simulink model "ALKEC_smlk"  (R2015b)
settings: Solver=VariableStepAuto  SolverMode=SingleTasking  StartTime=0.0  StopTime=1000  MaxStep=1  MinStep=0.0001  RelTol=1e-3
values from neighbouring files (symbols this model uses):
  A_cell = 0.25    [ALKEC_begin.m]
  c_cw = 4.18e03    (= 4180)    [ALKEC_cellstack.m]    (also in ALKEC_data.m)
  C_th = 625e03    (= 625000)    [ALKEC_data.m]
  DeltaP = (p_an - p_atm) / eta_p    [ALKEC_data.m]
  eta_ACDC = 0.95    [ALKEC_data.m]
  F = 96485    [ALKEC_begin.m]
  f1 = 2.50    (= 2.5)    [ALKEC_data.m]
  f2 = 0.97    [ALKEC_data.m]
  h_cond = 250    [ALKEC_data.m]
  h_conv = 0.97    [ALKEC_data.m]
  m_cw = 0.0850    (= 0.085)    [ALKEC_cellstack.m]    (also in ALKEC_data.m = 0.25)
  M_H2 = 2.01588    [ALKEC_cellstack.m]    (also in ALKEC_data.m)
  M_H2O = 18.01528    [ALKEC_cellstack.m]    (also in ALKEC_data.m)
  M_O2 = 31.9988    [ALKEC_cellstack.m]    (also in ALKEC_data.m)
  N_cell = 90    [ALKEC_begin.m]
  P_gamma = 2.5e03    (= 2500)    [ALKEC_data.m]
  p_H2avg = (p_H2in + p_H2out) / 2    [ALKEC_data.m]
  p_H2Oavg = (p_H2Oin + p_H2Oout) / 2    [ALKEC_data.m]
  p_O2avg = (p_O2in + p_O2out) / 2    [ALKEC_data.m]
  R = 8.314    [ALKEC_begin.m]
  r1 = 3.53855e-04    (= 0.000353855)    [ALKEC_data.m]
  r2 = -3.02150e-06    (= -3.0215e-06)    [ALKEC_data.m]
  R_th = 0.167    [ALKEC_data.m]
  s = 0.22396    [ALKEC_data.m]
  T = 80 + 273.15    (= 353.15)    [ALKEC_begin.m]
  T0 = T_a    [ALKEC_data.m]
  t1 = 2.73093    [ALKEC_data.m]
  t2 = -2.40447e02    (= -240.447)    [ALKEC_data.m]
  t3 = 5.99576e03    (= 5995.76)    [ALKEC_data.m]
  T_a = 25    [ALKEC_begin.m]
  T_amb = 25    [ALKEC_begin.m]    (also in ALKEC_data.m = T_a + 273.15)
  T_cwin = 20 + 0    (= 20)    [ALKEC_cellstack.m]    (also in ALKEC_data.m)
  T_des = T - 273.15    [ALKEC_data.m]
  tau_E = 2.00    (= 2)    [ALKEC_data.m]
  tau_p = 0.5    [ALKEC_data.m]
  tau_th = C_th * R_th    [ALKEC_cellstack.m]    (also in ALKEC_data.m = 104375)
  U = polyval(polU, I(1))    [ALKEC_data.m]
  v_H2 = 0.08988e03    (= 89.88)    [ALKEC_cellstack.m]    (also in ALKEC_data.m)
  v_H240 = 3.1777e03    (= 3177.7)    [ALKEC_data.m]
  v_H2O = 999.97e03    (= 999970)    [ALKEC_cellstack.m]    (also in ALKEC_data.m = 999700)
  v_O2 = 1.308e03    (= 1308)    [ALKEC_cellstack.m]    (also in ALKEC_data.m)
  v_O240 = 52.876e03    (= 52876)    [ALKEC_data.m]
  V_tn = 1.48    [ALKEC_cellstack.m]    (also in ALKEC_data.m)
  VS_H2 = 40    [ALKEC_data.m]
  VS_O2 = 20    [ALKEC_data.m]
  zeta = 1    [ALKEC_data.m]
undefined symbols (not defined in the file or in its folder): magnitude
settings Model: Creator=gapaolo  LastModifiedBy=gapaolo
settings DataIOCC: SaveFormat=Array
settings OptimizationCC: BlockReduction=off  BooleanDataType=off
settings DebuggingCC: AlgebraicLoopMsg=none  SaveWithParameterizedLinksMsg=none  UnderspecifiedInitializationDetection=Classic  MergeDetectMultiDrivingBlocksExec=none  SignalResolutionControl=TryResolveAllWithWarning
settings HardwareCC: ProdBitPerPointer=32  ProdLargestAtomicFloat=None  ProdIntDivRoundTo=Undefined  ProdEndianess=Unspecified  ProdWordSize=32  ProdHWDeviceType=32-bit Generic  TargetUnknown=on
settings GRTTargetCC: GeneratePreprocessorConditionals=Disable all
settings ConfigComp: CovModelRefEnable=Off  CovSFcnEnable=off

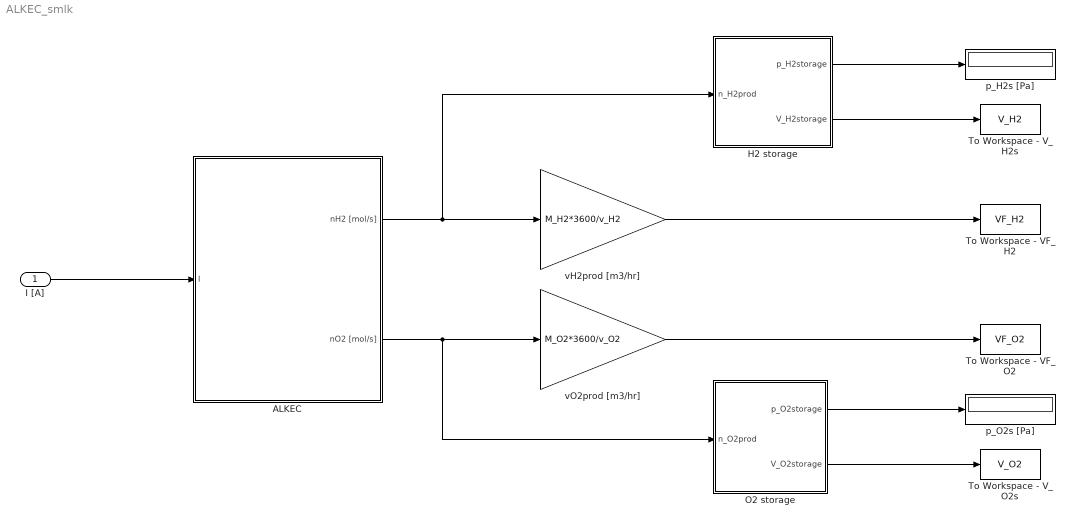
== system ALKEC_smlk ==
  I [A] : Inport
  ALKEC : Subsystem
  H2 storage : Subsystem
  O2 storage : Subsystem
  To Workspace - VF_H2 : ToWorkspace  VariableName=VF_H2  SaveFormat=Timeseries  SampleTime=-1
  To Workspace - VF_O2 : ToWorkspace  VariableName=VF_O2  SaveFormat=Timeseries  SampleTime=-1
  To Workspace - V_H2s : ToWorkspace  VariableName=V_H2  SaveFormat=Timeseries  SampleTime=-1
  To Workspace - V_O2s : ToWorkspace  VariableName=V_O2  SaveFormat=Timeseries  SampleTime=-1
  p_H2s [Pa] : Display
  p_O2s [Pa] : Display
  vH2prod [m3/hr] : Gain  Gain=M_H2*3600/v_H2
  vO2prod [m3/hr] : Gain  Gain=M_O2*3600/v_O2
  wires:
  I [A]/1 -> ALKEC/1(I)
  H2 storage/1(p_H2storage) -> p_H2s [Pa]/1
  ALKEC/2(nO2 [mol/s]) -> O2 storage/1(n_O2prod), vO2prod [m3/hr]/1
  O2 storage/1(p_O2storage) -> p_O2s [Pa]/1
  H2 storage/2(V_H2storage) -> To Workspace - V_H2s/1
  O2 storage/2(V_O2storage) -> To Workspace - V_O2s/1
  vH2prod [m3/hr]/1 -> To Workspace - VF_H2/1
  vO2prod [m3/hr]/1 -> To Workspace - VF_O2/1
  ALKEC/1(nH2 [mol/s]) -> H2 storage/1(n_H2prod), vH2prod [m3/hr]/1

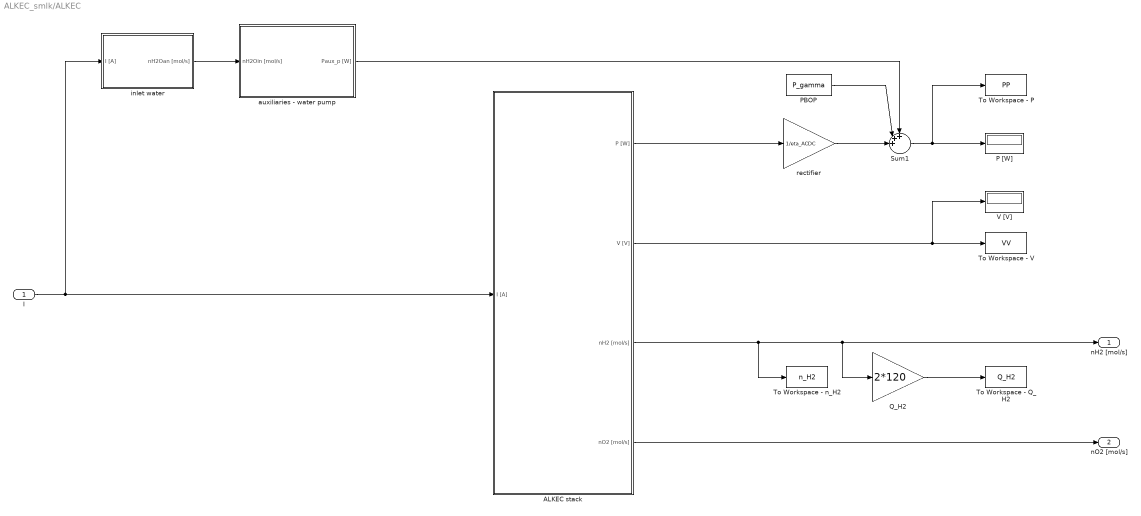
== system ALKEC_smlk/ALKEC ==
  I : Inport
  ALKEC stack : Subsystem
  P [W] : Display
  PBOP : Constant  Value=P_gamma
  Q_H2 : Gain  Gain=2*120
  Sum1 : Sum  Inputs=+++||
  To Workspace - P : ToWorkspace  VariableName=PP  SaveFormat=Timeseries  SampleTime=-1
  To Workspace - Q_H2 : ToWorkspace  VariableName=Q_H2  SaveFormat=Timeseries  SampleTime=-1
  To Workspace - V : ToWorkspace  VariableName=VV  SaveFormat=Timeseries  SampleTime=-1
  To Workspace - n_H2 : ToWorkspace  VariableName=n_H2  SaveFormat=Timeseries  SampleTime=-1
  V [V] : Display
  auxiliaries - water pump : Subsystem
  inlet water : Subsystem
  rectifier : Gain  Gain=1/eta_ACDC
  nH2 [mol/s] : Outport
  nO2 [mol/s] : Outport  Port=2
  wires:
  ALKEC stack/2(V [V]) -> To Workspace - V/1, V [V]/1
  I/1 -> inlet water/1(I [A]), ALKEC stack/1(I [A])
  ALKEC stack/1(P [W]) -> rectifier/1
  inlet water/1("nH2Oan [mol/s] ") -> auxiliaries - water pump/1(nH2Oin [mol/s])
  rectifier/1 -> Sum1/3
  Sum1/1 -> To Workspace - P/1, P [W]/1
  PBOP/1 -> Sum1/2
  auxiliaries - water pump/1(Paux_p [W]) -> Sum1/1
  ALKEC stack/4(nO2 [mol/s]) -> nO2 [mol/s]/1
  ALKEC stack/3(nH2 [mol/s]) -> To Workspace - n_H2/1, Q_H2/1, nH2 [mol/s]/1
  Q_H2/1 -> To Workspace - Q_H2/1

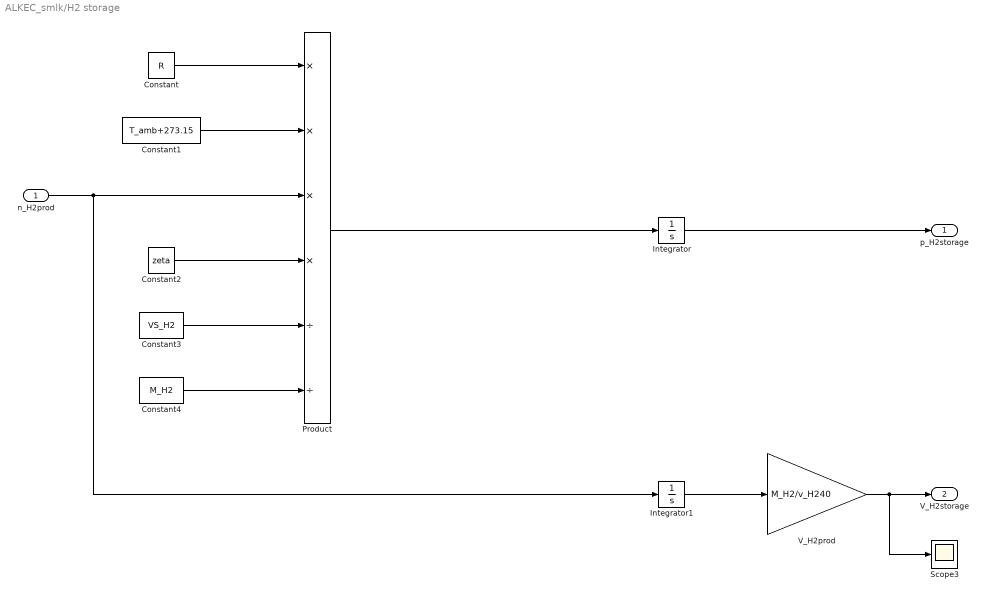
== system ALKEC_smlk/H2 storage ==
  n_H2prod : Inport
  Constant : Constant  Value=R
  Constant1 : Constant  Value=T_amb+273.15
  Constant2 : Constant  Value=zeta
  Constant3 : Constant  Value=VS_H2
  Constant4 : Constant  Value=M_H2
  Integrator : Integrator  InitialCondition=101325
  Integrator1 : Integrator
  Product : Product  Inputs=****//
  Scope3 : Scope
  V_H2prod : Gain  Gain=M_H2/v_H240
  p_H2storage : Outport
  V_H2storage : Outport  Port=2
  wires:
  n_H2prod/1 -> Integrator1/1, Product/3
  Constant/1 -> Product/1
  Constant1/1 -> Product/2
  Constant2/1 -> Product/4
  Constant3/1 -> Product/5
  Constant4/1 -> Product/6
  Product/1 -> Integrator/1
  Integrator/1 -> p_H2storage/1
  Integrator1/1 -> V_H2prod/1
  V_H2prod/1 -> Scope3/1, V_H2storage/1

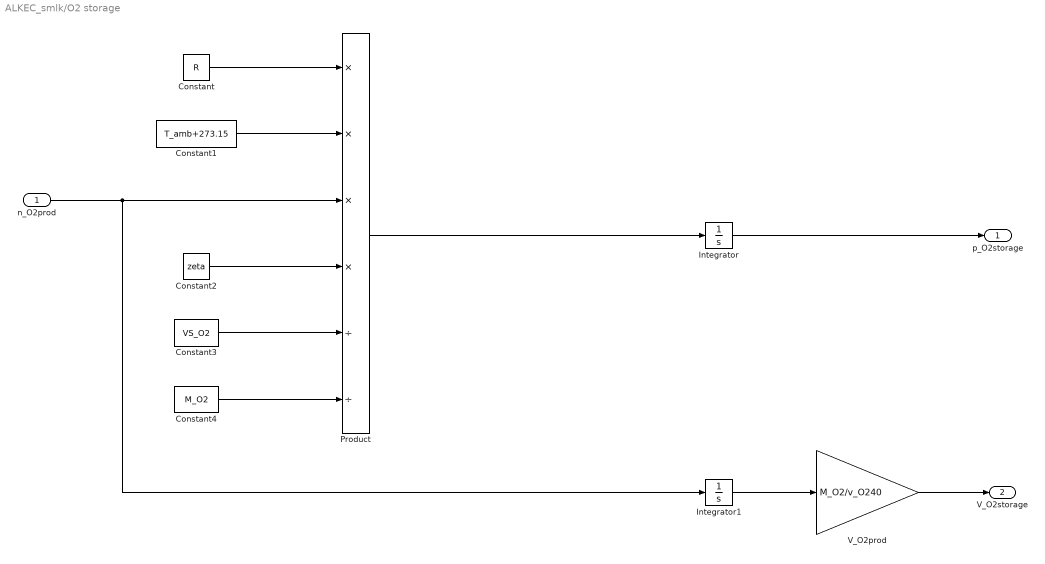
== system ALKEC_smlk/O2 storage ==
  n_O2prod : Inport
  Constant : Constant  Value=R
  Constant1 : Constant  Value=T_amb+273.15
  Constant2 : Constant  Value=zeta
  Constant3 : Constant  Value=VS_O2
  Constant4 : Constant  Value=M_O2
  Integrator : Integrator  InitialCondition=101325
  Integrator1 : Integrator
  Product : Product  Inputs=****//
  V_O2prod : Gain  Gain=M_O2/v_O240
  p_O2storage : Outport
  V_O2storage : Outport  Port=2
  wires:
  n_O2prod/1 -> Integrator1/1, Product/3
  Constant/1 -> Product/1
  Constant1/1 -> Product/2
  Constant2/1 -> Product/4
  Constant3/1 -> Product/5
  Constant4/1 -> Product/6
  Product/1 -> Integrator/1
  Integrator/1 -> p_O2storage/1
  Integrator1/1 -> V_O2prod/1
  V_O2prod/1 -> V_O2storage/1

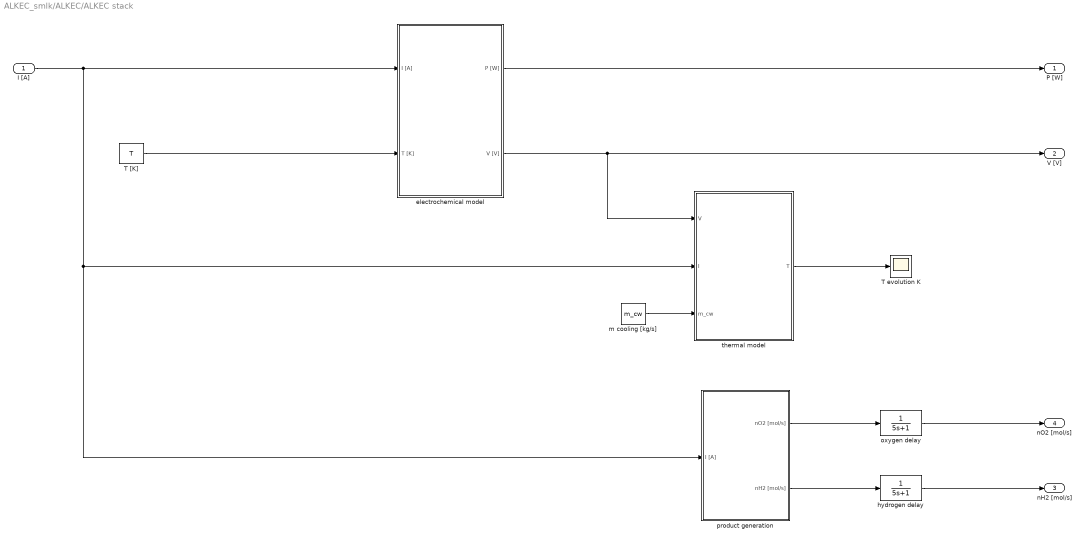
== system ALKEC_smlk/ALKEC/ALKEC stack ==
  I [A] : Inport
  T [K] : Constant  Value=T
  T evolution K : Scope
  electrochemical model : Subsystem
  hydrogen delay : TransferFcn  Denominator=[5 1]
  m cooling [kg/s] : Constant  Value=m_cw
  oxygen delay : TransferFcn  Denominator=[5 1]
  product generation : Subsystem
  thermal model : Subsystem
  P [W] : Outport
  V [V] : Outport  Port=2
  nH2 [mol/s] : Outport  Port=3
  nO2 [mol/s] : Outport  Port=4
  wires:
  m cooling [kg/s]/1 -> thermal model/3(m_cw)
  electrochemical model/2(V [V]) -> V [V]/1, thermal model/1(V)
  thermal model/1(T) -> T evolution K/1
  electrochemical model/1(P [W]) -> P [W]/1
  I [A]/1 -> product generation/1(I [A]), thermal model/2(I), electrochemical model/1(I [A])
  T [K]/1 -> electrochemical model/2(T [K])
  oxygen delay/1 -> nO2 [mol/s]/1
  hydrogen delay/1 -> nH2 [mol/s]/1
  product generation/1(nO2 [mol/s]) -> oxygen delay/1
  product generation/2(nH2 [mol/s]) -> hydrogen delay/1

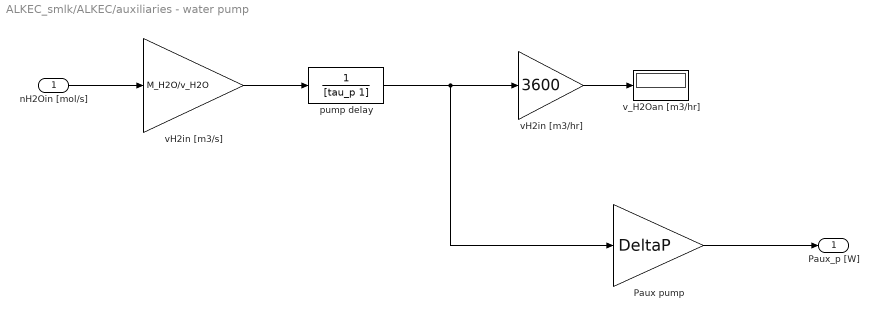
== system ALKEC_smlk/ALKEC/auxiliaries - water pump ==
  nH2Oin [mol/s] : Inport
  Paux pump : Gain  Gain=DeltaP
  pump delay : TransferFcn  Denominator=[tau_p 1]
  vH2in [m3/hr] : Gain  Gain=3600
  vH2in [m3/s] : Gain  Gain=M_H2O/v_H2O
  v_H2Oan [m3/hr] : Display
  Paux_p [W] : Outport
  wires:
  vH2in [m3/s]/1 -> pump delay/1
  vH2in [m3/hr]/1 -> v_H2Oan [m3/hr]/1
  Paux pump/1 -> Paux_p [W]/1
  nH2Oin [mol/s]/1 -> vH2in [m3/s]/1
  pump delay/1 -> vH2in [m3/hr]/1, Paux pump/1

== system ALKEC_smlk/ALKEC/inlet water ==
  I [A] : Inport
  Faraday efficiency : Subsystem
  I*eta_F : Product
  n_H2Ocons1 : Gain  Gain=N_cell/(2*F*U)
  "nH2Oan [mol/s] " : Outport
  wires:
  Faraday efficiency/2(I [A]) -> I*eta_F/2
  Faraday efficiency/1(eta_F) -> I*eta_F/1
  I*eta_F/1 -> n_H2Ocons1/1
  n_H2Ocons1/1 -> "nH2Oan [mol/s] "/1
  I [A]/1 -> Faraday efficiency/1(I)

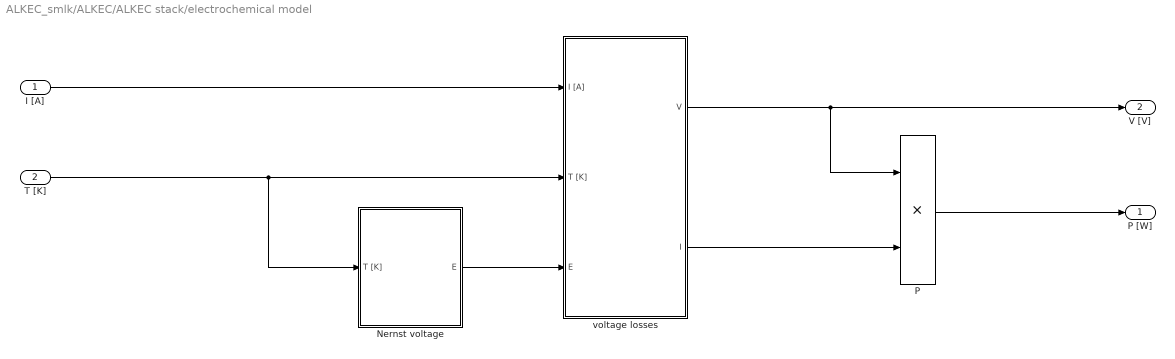
== system ALKEC_smlk/ALKEC/ALKEC stack/electrochemical model ==
  I [A] : Inport
  T [K] : Inport  Port=2
  Nernst voltage : Subsystem
  P : Product
  "voltage losses " : Subsystem
  P [W] : Outport
  V [V] : Outport  Port=2
  wires:
  I [A]/1 -> "voltage losses "/1("I [A] ")
  "voltage losses "/1(V) -> P/1, V [V]/1
  P/1 -> P [W]/1
  T [K]/1 -> "voltage losses "/2(T [K]), Nernst voltage/1(T [K])
  "voltage losses "/2(I) -> P/2
  Nernst voltage/1(E) -> "voltage losses "/3(E)

== system ALKEC_smlk/ALKEC/ALKEC stack/product generation ==
  I [A] : Inport
  Faraday efficiency : Subsystem
  I*eta_F : Product
  n_H2 : Gain  Gain=N_cell/(2*F)
  n_O2 : Gain  Gain=N_cell/(4*F)
  nO2 [mol/s] : Outport
  nH2 [mol/s] : Outport  Port=2
  wires:
  n_H2/1 -> nH2 [mol/s]/1
  n_O2/1 -> nO2 [mol/s]/1
  I [A]/1 -> Faraday efficiency/1(I)
  Faraday efficiency/2(I [A]) -> I*eta_F/2
  Faraday efficiency/1(eta_F) -> I*eta_F/1
  I*eta_F/1 -> n_O2/1, n_H2/1

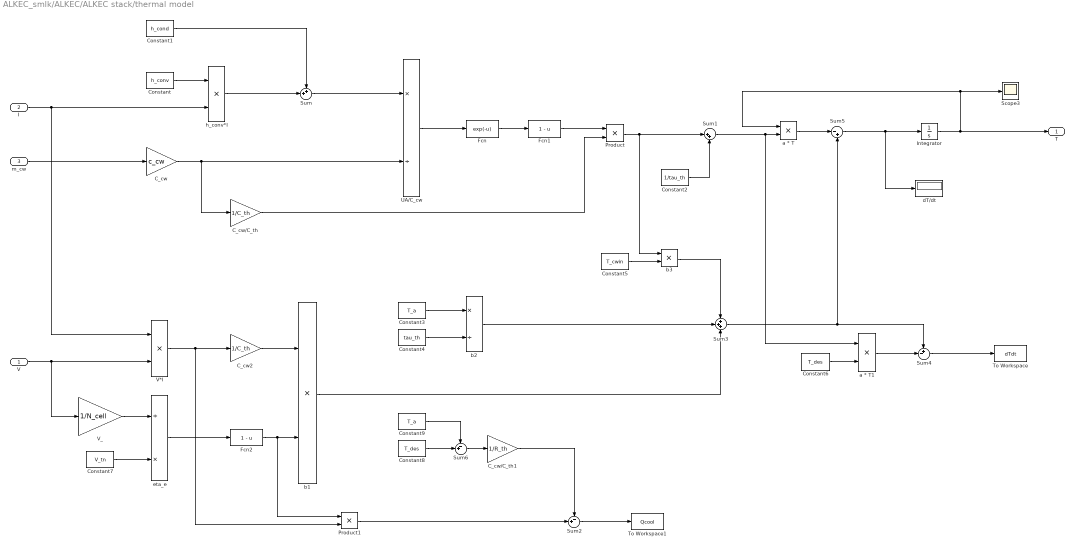
== system ALKEC_smlk/ALKEC/ALKEC stack/thermal model ==
  V : Inport
  I : Inport  Port=2
  m_cw : Inport  Port=3
  C_cw : Gain  Gain=c_cw
  C_cw/C_th : Gain  Gain=1/C_th
  C_cw/C_th1 : Gain  Gain=1/R_th
  C_cw2 : Gain  Gain=1/C_th
  Constant : Constant  Value=h_conv
  Constant1 : Constant  Value=h_cond
  Constant2 : Constant  Value=1/tau_th
  Constant3 : Constant  Value=T_a
  Constant4 : Constant  Value=tau_th
  Constant5 : Constant  Value=T_cwin
  Constant6 : Constant  Value=T_des
  Constant7 : Constant  Value=V_tn
  Constant8 : Constant  Value=T_des
  Constant9 : Constant  Value=T_a
  Fcn : Fcn  Expr=exp(-u)
  Fcn1 : Fcn  Expr=1 - u
  Fcn2 : Fcn  Expr=1 - u
  Integrator : Integrator  InitialCondition=T0
  Product : Product
  Product1 : Product
  Scope3 : Scope
  Sum : Sum  Inputs=++|
  Sum1 : Sum  Inputs=|++
  Sum2 : Sum  Inputs=-+|
  Sum3 : Sum  Inputs=+++
  Sum4 : Sum  Inputs=+-|
  Sum5 : Sum  Inputs=|-+
  Sum6 : Sum  Inputs=-+|
  To Workspace : ToWorkspace  VariableName=dTdt  SaveFormat=Timeseries  SampleTime=-1
  To Workspace1 : ToWorkspace  VariableName=Qcool  SaveFormat=Timeseries  SampleTime=-1
  UA/C_cw : Product  Inputs=*/
  V*I : Product
  V_ : Gain  Gain=1/N_cell
  a * T : Product
  a * T1 : Product
  b1 : Product
  b2 : Product  Inputs=*/
  b3 : Product
  dT/dt : Display
  eta_e : Product  Inputs=/*
  h_conv*I : Product
  T : Outport
  wires:
  I/1 -> V*I/1, h_conv*I/2
  Constant/1 -> h_conv*I/1
  h_conv*I/1 -> Sum/2
  Constant1/1 -> Sum/1
  Sum/1 -> UA/C_cw/1
  m_cw/1 -> C_cw/1
  UA/C_cw/1 -> Fcn/1
  Fcn/1 -> Fcn1/1
  C_cw/1 -> UA/C_cw/2, C_cw/C_th/1
  Fcn1/1 -> Product/1
  C_cw/C_th/1 -> Product/2
  Product/1 -> b3/1, Sum1/1
  Constant2/1 -> Sum1/2
  C_cw2/1 -> b1/1
  Constant3/1 -> b2/1
  Constant4/1 -> b2/2
  Constant5/1 -> b3/2
  b3/1 -> Sum3/1
  b2/1 -> Sum3/2
  V_/1 -> eta_e/1
  Constant7/1 -> eta_e/2
  eta_e/1 -> Fcn2/1
  Sum5/1 -> dT/dt/1, Integrator/1
  a * T/1 -> Sum5/1
  Sum1/1 -> a * T1/1, a * T/2
  Integrator/1 -> a * T/1, Scope3/1, T/1
  b1/1 -> Sum3/3
  Sum3/1 -> Sum4/1, Sum5/2
  Constant6/1 -> a * T1/2
  Sum4/1 -> To Workspace/1
  a * T1/1 -> Sum4/2
  Product1/1 -> Sum2/2
  Constant8/1 -> Sum6/2
  Constant9/1 -> Sum6/1
  Sum6/1 -> C_cw/C_th1/1
  C_cw/C_th1/1 -> Sum2/1
  Sum2/1 -> To Workspace1/1
  V*I/1 -> Product1/2, C_cw2/1
  Fcn2/1 -> Product1/1, b1/2
  V/1 -> V*I/2, V_/1

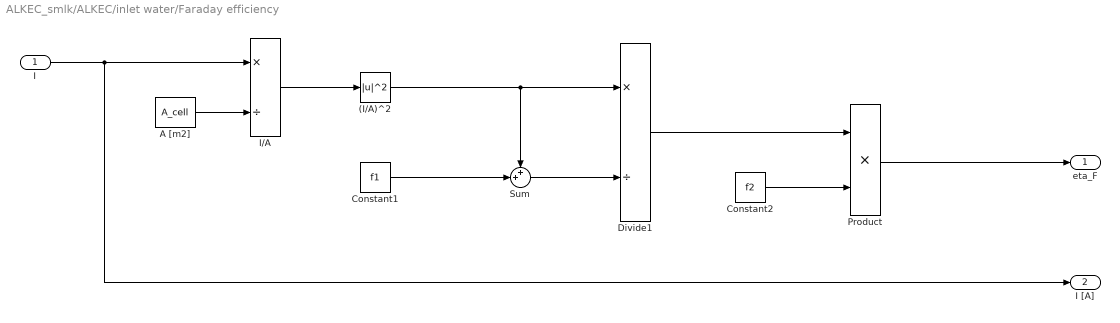
== system ALKEC_smlk/ALKEC/inlet water/Faraday efficiency ==
  I : Inport
  (I/A)^2 : Math  Operator=magnitude^2  SaturateOnIntegerOverflow=on
  A [m2] : Constant  Value=A_cell
  Constant1 : Constant  Value=f1
  Constant2 : Constant  Value=f2
  Divide1 : Product  Inputs=*/
  I/A : Product  Inputs=*/
  Product : Product
  Sum : Sum  Inputs=++|
  eta_F : Outport
  I [A] : Outport  Port=2
  wires:
  A [m2]/1 -> I/A/2
  I/1 -> I [A]/1, I/A/1
  I/A/1 -> (I/A)^2/1
  (I/A)^2/1 -> Sum/1, Divide1/1
  Constant1/1 -> Sum/2
  Sum/1 -> Divide1/2
  Divide1/1 -> Product/1
  Constant2/1 -> Product/2
  Product/1 -> eta_F/1

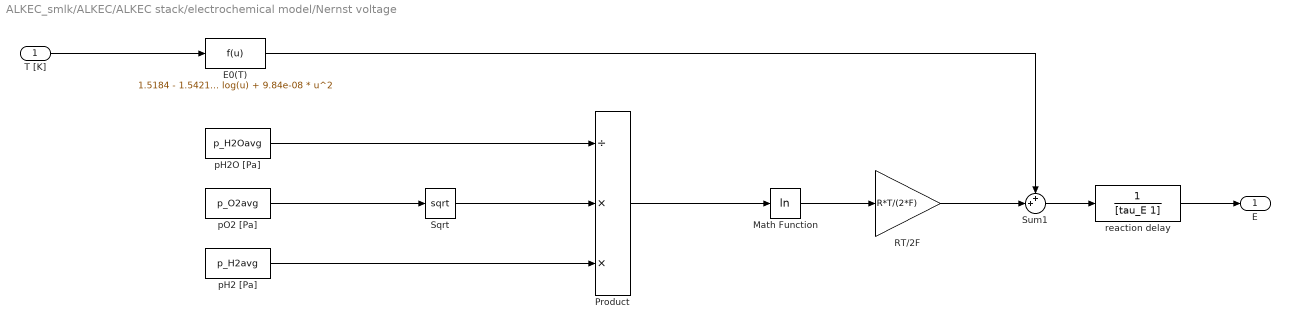
== system ALKEC_smlk/ALKEC/ALKEC stack/electrochemical model/Nernst voltage ==
  T [K] : Inport
  E0(T) : Fcn  Expr=1.5184 - 1.5421e-03 * u + 9.523e-05 * u * log(u) + 9.84e-08 * u^2
  Math Function : Math  Operator=log  SaturateOnIntegerOverflow=on
  Product : Product  Inputs=/**
  RT/2F : Gain  Gain=R*T/(2*F)
  Sqrt : Sqrt  SaturateOnIntegerOverflow=on
  Sum1 : Sum  Inputs=++|
  pH2 [Pa] : Constant  Value=p_H2avg
  pH2O [Pa] : Constant  Value=p_H2Oavg
  pO2 [Pa] : Constant  Value=p_O2avg
  reaction delay : TransferFcn  Denominator=[tau_E 1]
  E : Outport
  wires:
  RT/2F/1 -> Sum1/2
  E0(T)/1 -> Sum1/1
  Sum1/1 -> reaction delay/1
  Sqrt/1 -> Product/2
  Product/1 -> Math Function/1
  Math Function/1 -> RT/2F/1
  T [K]/1 -> E0(T)/1
  pH2O [Pa]/1 -> Product/1
  pH2 [Pa]/1 -> Product/3
  pO2 [Pa]/1 -> Sqrt/1
  reaction delay/1 -> E/1

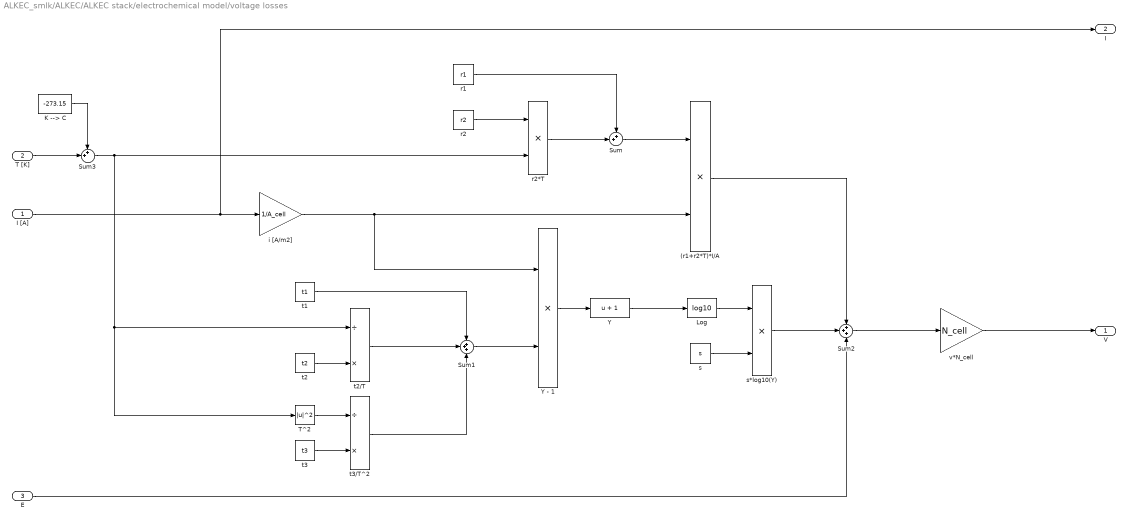
== system ALKEC_smlk/ALKEC/ALKEC stack/electrochemical model/voltage losses  ==
  "I [A] " : Inport
  T [K] : Inport  Port=2
  E : Inport  Port=3
  (r1+r2*T)*I/A : Product  Inputs=**
  K --> C : Constant  Value=-273.15
  Log : Math  Operator=log10  SaturateOnIntegerOverflow=on
  Sum : Sum  Inputs=++|
  Sum1 : Sum  Inputs=+++
  Sum2 : Sum  Inputs=+++
  Sum3 : Sum  Inputs=++|
  T^2 : Math  Operator=magnitude^2  SaturateOnIntegerOverflow=on
  Y : Fcn  Expr=u + 1
  Y - 1 : Product  Inputs=**
  i [A/m2] : Gain  Gain=1/A_cell
  r1 : Constant  Value=r1
  r2 : Constant  Value=r2
  r2*T : Product  Inputs=**
  s : Constant  Value=s
  s*log10(Y) : Product  Inputs=**
  t1 : Constant  Value=t1
  t2 : Constant  Value=t2
  t2/T : Product  Inputs=/*
  t3 : Constant  Value=t3
  t3/T^2 : Product  Inputs=/*
  v*N_cell : Gain  Gain=N_cell
  V : Outport
  I : Outport  Port=2
  wires:
  E/1 -> Sum2/3
  "I [A] "/1 -> I/1, i [A/m2]/1
  v*N_cell/1 -> V/1
  r2/1 -> r2*T/1
  r2*T/1 -> Sum/2
  r1/1 -> Sum/1
  Sum/1 -> (r1+r2*T)*I/A/1
  i [A/m2]/1 -> Y - 1/1, (r1+r2*T)*I/A/2
  t2/1 -> t2/T/2
  t3/1 -> t3/T^2/2
  t2/T/1 -> Sum1/2
  t1/1 -> Sum1/1
  t3/T^2/1 -> Sum1/3
  Y - 1/1 -> Y/1
  Y/1 -> Log/1
  s/1 -> s*log10(Y)/2
  Log/1 -> s*log10(Y)/1
  s*log10(Y)/1 -> Sum2/2
  (r1+r2*T)*I/A/1 -> Sum2/1
  Sum2/1 -> v*N_cell/1
  T^2/1 -> t3/T^2/1
  Sum1/1 -> Y - 1/2
  Sum3/1 -> T^2/1, t2/T/1, r2*T/2
  T [K]/1 -> Sum3/2
  K --> C/1 -> Sum3/1

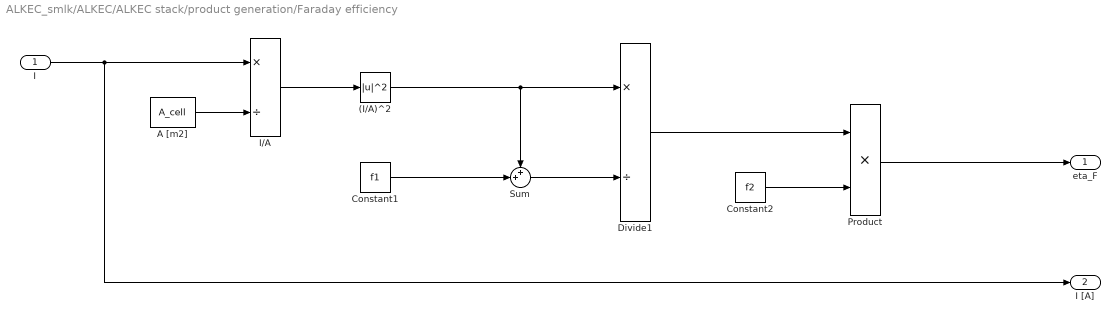
== system ALKEC_smlk/ALKEC/ALKEC stack/product generation/Faraday efficiency ==
  I : Inport
  (I/A)^2 : Math  Operator=magnitude^2  SaturateOnIntegerOverflow=on
  A [m2] : Constant  Value=A_cell
  Constant1 : Constant  Value=f1
  Constant2 : Constant  Value=f2
  Divide1 : Product  Inputs=*/
  I/A : Product  Inputs=*/
  Product : Product
  Sum : Sum  Inputs=++|
  eta_F : Outport
  I [A] : Outport  Port=2
  wires:
  A [m2]/1 -> I/A/2
  I/1 -> I [A]/1, I/A/1
  I/A/1 -> (I/A)^2/1
  (I/A)^2/1 -> Sum/1, Divide1/1
  Constant1/1 -> Sum/2
  Sum/1 -> Divide1/2
  Divide1/1 -> Product/1
  Constant2/1 -> Product/2
  Product/1 -> eta_F/1
